simulink model "mrefrobotarm_previous_y_previous_u_previous_ref_cex_2"  (R2018b)
settings: Solver=FixedStepAuto  StartTime=0.0  StopTime=20  RelTol=1e-3  AbsTol=1e-6
undefined symbols (not defined in the file or in its folder): cc, options
libraries: neural x462, simulink x2
(part 6 of 18)

== system mrefrobotarm_previous_y_previous_u_previous_ref_cex_2/Feed-Forward Neural Network1/Layer 3/Delays 1 ==
  "p{3}" : Inport  PortDimensions=30
      mask Display: e = 0.06;c1 = [120 230 180]/255;c2 = ([120 230 180]+0)/(256+128);c3 = ([120 230 180]+128)/(256+128);patch([0 1 1 0],[0 0 1 1],c1);patch([0 1 1 1-e 1-e 0+e],[0 0 1 1-e 0+e 0+e],c2);patch([0 0 1 1-e 0+e 0+e],[0 1 1 1-e 1-e 0+e],c3);plot([0 1 1 0 0],[0 0 1 1 0]);
  mux : Mux  Inputs=1
      mask Display: e = 0.06;c1 = [120 150 230]/255;c2 = ([120 150 230]+0)/383;c3 = ([120 150 230]+128)/383;patch([0 1 1 0],[0 0 1 1],c1);patch([0 1 1 1-e 1-e 0+e],[0 0 1 1-e 0+e 0+e],c2);patch([0 0 1 1-e 0+e 0+e],[0 1 1 1-e 1-e 0+e],c3);plot([0 1 1 0 0],[0 0 1 1 0]);disp('Mux')
  "pd{3,2}" : Outport
      mask Display: e = 0.06;c1 = [120 230 180]/255;c2 = ([120 230 180]+0)/(256+128);c3 = ([120 230 180]+128)/(256+128);patch([0 1 1 0],[0 0 1 1],c1);patch([0 1 1 1-e 1-e 0+e],[0 0 1 1-e 0+e 0+e],c2);patch([0 0 1 1-e 0+e 0+e],[0 1 1 1-e 1-e 0+e],c3);plot([0 1 1 0 0],[0 0 1 1 0]);
  wires:
  "p{3}"/1 -> mux/1
  mux/1 -> "pd{3,2}"/1

== system mrefrobotarm_previous_y_previous_u_previous_ref_cex_2/Feed-Forward Neural Network1/Layer 3/LW{3,2} ==
  "ad{3,2}" : Inport  PortDimensions=30
      mask Display: e = 0.06;c1 = [120 230 180]/255;c2 = ([120 230 180]+0)/(256+128);c3 = ([120 230 180]+128)/(256+128);patch([0 1 1 0],[0 0 1 1],c1);patch([0 1 1 1-e 1-e 0+e],[0 0 1 1-e 0+e 0+e],c2);patch([0 0 1 1-e 0+e 0+e],[0 1 1 1-e 1-e 0+e],c3);plot([0 1 1 0 0],[0 0 1 1 0]);
  "IW{3,2}(1,:)'" : Constant  Value=[0.245566465926212396109207247718586586415767669677734375;-0.56322081322037842454619749332778155803680419921875;-0.28991010367060410235495737651945091784000396728515625;0.3869683333504421174353637979947961866855621337890625;0.496517765752567064030387200546101666986942291259765625;-0.320943780837954883988771825897856615483760833740234375;0.0286370319336148211608605862465992686338722705841064453125;-0.15395906619913668489374458658858202397823333740234375;0.51493301451079076525019218024681322276592254638671875;-0.026941881639260277514491548345176852308213710784912109375;-0.05589778476223307424053388103857287205755710601806640625;0.1600136141061642980343293629630352370440959930419921875;-0.2212967731759021561277478440388222225010395050048828125;-0.168090459815553538991395043922238983213901519775390625;-0.4615503546136172641212169764912687242031097412109375;-0.60839853859597503582534727684105746448040008544921875;0.1504483327033876438605375369661487638950347900390625;-0.4073407234202310878146136019495315849781036376953125;0.331316055045982882365507293798145838081836700439453125;-0.1747391852843100945591459094430319964885711669921875;-0.19591165143500910428286942988052032887935638427734375;0.1816474984983245388736605718804639764130115509033203125;0.3783772749804861224021124144201166927814483642578125;0.046857186277910960192638611943038995377719402313232421875;-0.292883801455053660589555875048972666263580322265625;0.480373124807368323541112431485089473426342010498046875;-0.0158594532240923617727457184400918777100741863250732421875;-0.0228072195102398851684899483416302246041595935821533203125;-0.55934110245892210144802447757683694362640380859375;0.2422309302660256846717601320051471702754497528076171875]
      mask Display: e = 0.06;c1 = [120 150 230]/255;c2 = ([120 150 230]+0)/383;c3 = ([120 150 230]+128)/383;patch([0 1 1 0],[0 0 1 1],c1);patch([0 1 1 1-e 1-e 0+e],[0 0 1 1-e 0+e 0+e],c2);patch([0 0 1 1-e 0+e 0+e],[0 1 1 1-e 1-e 0+e],c3);plot([0 1 1 0 0],[0 0 1 1 0]);disp('weights');
  Mux : Mux  Inputs=1
      mask Display: e = 0.06;c1 = [120 150 230]/255;c2 = ([120 150 230]+0)/383;c3 = ([120 150 230]+128)/383;patch([0 1 1 0],[0 0 1 1],c1);patch([0 1 1 1-e 1-e 0+e],[0 0 1 1-e 0+e 0+e],c2);patch([0 0 1 1-e 0+e 0+e],[0 1 1 1-e 1-e 0+e],c3);plot([0 1 1 0 0],[0 0 1 1 0]);disp('Mux');
  dotprod1 : neural/Weight Functions/dotprod
  "lz{3,2}" : Outport
      mask Display: e = 0.06;c1 = [120 230 180]/255;c2 = ([120 230 180]+0)/(256+128);c3 = ([120 230 180]+128)/(256+128);patch([0 1 1 0],[0 0 1 1],c1);patch([0 1 1 1-e 1-e 0+e],[0 0 1 1-e 0+e 0+e],c2);patch([0 0 1 1-e 0+e 0+e],[0 1 1 1-e 1-e 0+e],c3);plot([0 1 1 0 0],[0 0 1 1 0]);
  wires:
  "IW{3,2}(1,:)'"/1 -> dotprod1/1
  "ad{3,2}"/1 -> dotprod1/2
  dotprod1/1 -> Mux/1
  Mux/1 -> "lz{3,2}"/1

== system mrefrobotarm_previous_y_previous_u_previous_ref_cex_2/cex_m1/Layer 1/Delays 1 ==
  "p{1}" : Inport  PortDimensions=10
      mask Display: e = 0.06;c1 = [120 230 180]/255;c2 = ([120 230 180]+0)/(256+128);c3 = ([120 230 180]+128)/(256+128);patch([0 1 1 0],[0 0 1 1],c1);patch([0 1 1 1-e 1-e 0+e],[0 0 1 1-e 0+e 0+e],c2);patch([0 0 1 1-e 0+e 0+e],[0 1 1 1-e 1-e 0+e],c3);plot([0 1 1 0 0],[0 0 1 1 0]);
  mux : Mux  Inputs=1
      mask Display: e = 0.06;c1 = [120 150 230]/255;c2 = ([120 150 230]+0)/383;c3 = ([120 150 230]+128)/383;patch([0 1 1 0],[0 0 1 1],c1);patch([0 1 1 1-e 1-e 0+e],[0 0 1 1-e 0+e 0+e],c2);patch([0 0 1 1-e 0+e 0+e],[0 1 1 1-e 1-e 0+e],c3);plot([0 1 1 0 0],[0 0 1 1 0]);disp('Mux')
  "pd{1,1}" : Outport
      mask Display: e = 0.06;c1 = [120 230 180]/255;c2 = ([120 230 180]+0)/(256+128);c3 = ([120 230 180]+128)/(256+128);patch([0 1 1 0],[0 0 1 1],c1);patch([0 1 1 1-e 1-e 0+e],[0 0 1 1-e 0+e 0+e],c2);patch([0 0 1 1-e 0+e 0+e],[0 1 1 1-e 1-e 0+e],c3);plot([0 1 1 0 0],[0 0 1 1 0]);
  wires:
  "p{1}"/1 -> mux/1
  mux/1 -> "pd{1,1}"/1

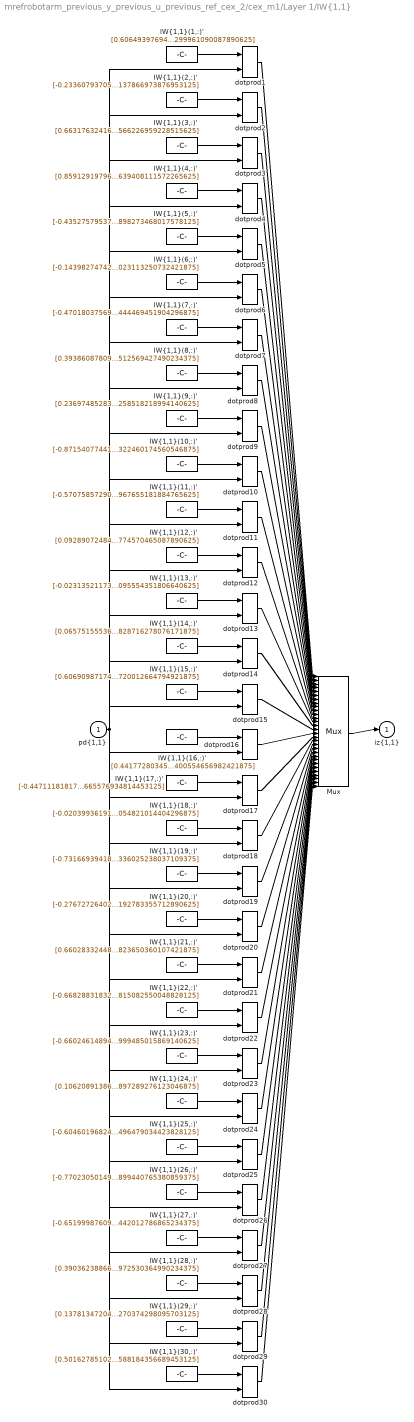
== system mrefrobotarm_previous_y_previous_u_previous_ref_cex_2/cex_m1/Layer 1/IW{1,1} ==
  "pd{1,1}" : Inport  PortDimensions=10
      mask Display: e = 0.06;c1 = [120 230 180]/255;c2 = ([120 230 180]+0)/(256+128);c3 = ([120 230 180]+128)/(256+128);patch([0 1 1 0],[0 0 1 1],c1);patch([0 1 1 1-e 1-e 0+e],[0 0 1 1-e 0+e 0+e],c2);patch([0 0 1 1-e 0+e 0+e],[0 1 1 1-e 1-e 0+e],c3);plot([0 1 1 0 0],[0 0 1 1 0]);
  "IW{1,1}(1,:)'" : Constant  Value=[0.606493976942152013265285859233699738979339599609375;0.300870328462947533854077164505724795162677764892578125;0.58384608162362194860861563938669860363006591796875;-0.183702727789528175161848366769845597445964813232421875;-0.256826958227045765159601842242409475147724151611328125;-0.11957272826138511112592510698959813453257083892822265625;-0.94857591659136308859245900748646818101406097412109375;0.6791329614163685857164409753750078380107879638671875;-0.58145783774079229377917954479926265776157379150390625;0.78323377095806601122518486590706743299961090087890625]
      mask Display: e = 0.06;c1 = [120 150 230]/255;c2 = ([120 150 230]+0)/383;c3 = ([120 150 230]+128)/383;patch([0 1 1 0],[0 0 1 1],c1);patch([0 1 1 1-e 1-e 0+e],[0 0 1 1-e 0+e 0+e],c2);patch([0 0 1 1-e 0+e 0+e],[0 1 1 1-e 1-e 0+e],c3);plot([0 1 1 0 0],[0 0 1 1 0]);disp('Weights');
  "IW{1,1}(10,:)'" : Constant  Value=[-0.87154077441328325903668883256614208221435546875;1.049912196434298561342757238890044391155242919921875;0.27458172096172395182378522804356180131435394287109375;-0.711717329252754549173687337315641343593597412109375;0.27785454353788729964236381420050747692584991455078125;-0.0815691029770375386487302193927462212741374969482421875;0.23890314712288562848385709003196097910404205322265625;0.239853933232654858986876433846191503107547760009765625;-0.62431495878185250258951555224484764039516448974609375;-0.777991313273826090579632364097051322460174560546875]
      mask Display: e = 0.06;c1 = [120 150 230]/255;c2 = ([120 150 230]+0)/383;c3 = ([120 150 230]+128)/383;patch([0 1 1 0],[0 0 1 1],c1);patch([0 1 1 1-e 1-e 0+e],[0 0 1 1-e 0+e 0+e],c2);patch([0 0 1 1-e 0+e 0+e],[0 1 1 1-e 1-e 0+e],c3);plot([0 1 1 0 0],[0 0 1 1 0]);disp('Weights');
  "IW{1,1}(11,:)'" : Constant  Value=[-0.57075857290971854229866266905446536839008331298828125;0.9105044883497910301883848660509102046489715576171875;-0.0274634831225473614868537453048702445812523365020751953125;-0.254607299960154798146305665795807726681232452392578125;-0.2120219789851869596208899793055024929344654083251953125;-0.07760455330727596134909873626384069211781024932861328125;0.42068189247083986881392547729774378240108489990234375;-0.5132735800885883659105957121937535703182220458984375;-0.57046668147494450362700035839225165545940399169921875;-0.750017524258132173287094701663590967655181884765625]
      mask Display: e = 0.06;c1 = [120 150 230]/255;c2 = ([120 150 230]+0)/383;c3 = ([120 150 230]+128)/383;patch([0 1 1 0],[0 0 1 1],c1);patch([0 1 1 1-e 1-e 0+e],[0 0 1 1-e 0+e 0+e],c2);patch([0 0 1 1-e 0+e 0+e],[0 1 1 1-e 1-e 0+e],c3);plot([0 1 1 0 0],[0 0 1 1 0]);disp('Weights');
  "IW{1,1}(12,:)'" : Constant  Value=[0.09289072484482759073376456626647268421947956085205078125;-0.9326730997274779166872349378536455333232879638671875;-0.8047520255107321052179258913383819162845611572265625;-0.530309467610881934973576790071092545986175537109375;0.5676139588165167726430127004277892410755157470703125;-0.60426402156130032405911833848222158849239349365234375;0.416928927700072560202926297279191203415393829345703125;0.56024270477934645651174605518463067710399627685546875;0.130929582458561399871399544281302951276302337646484375;-0.45882086062754334765401154072606004774570465087890625]
      mask Display: e = 0.06;c1 = [120 150 230]/255;c2 = ([120 150 230]+0)/383;c3 = ([120 150 230]+128)/383;patch([0 1 1 0],[0 0 1 1],c1);patch([0 1 1 1-e 1-e 0+e],[0 0 1 1-e 0+e 0+e],c2);patch([0 0 1 1-e 0+e 0+e],[0 1 1 1-e 1-e 0+e],c3);plot([0 1 1 0 0],[0 0 1 1 0]);disp('Weights');
  "IW{1,1}(13,:)'" : Constant  Value=[-0.0231352117399873831449230721091225859709084033966064453125;-0.796505407556588718165357931866310536861419677734375;-0.5816665559413660702148263226263225078582763671875;-0.9505142528724146444574216729961335659027099609375;0.1164862638332339328517406329410732723772525787353515625;0.608926424961647949629650611313991248607635498046875;-0.257541098890456565673190425513894297182559967041015625;0.33512401139020220330877464220975525677204132080078125;0.03018497961469925050526086351965204812586307525634765625;-0.9364213635540326041706293835886754095554351806640625]
      mask Display: e = 0.06;c1 = [120 150 230]/255;c2 = ([120 150 230]+0)/383;c3 = ([120 150 230]+128)/383;patch([0 1 1 0],[0 0 1 1],c1);patch([0 1 1 1-e 1-e 0+e],[0 0 1 1-e 0+e 0+e],c2);patch([0 0 1 1-e 0+e 0+e],[0 1 1 1-e 1-e 0+e],c3);plot([0 1 1 0 0],[0 0 1 1 0]);disp('Weights');
  "IW{1,1}(14,:)'" : Constant  Value=[0.06575155536450284776694985566791729070246219635009765625;-0.99234351852335211940925319140660576522350311279296875;-0.0584833978458139114309233264066278934478759765625;0.157791463982731972048867419289308600127696990966796875;-0.208312265611119429298270233630319125950336456298828125;0.2878455117467508816986310193897224962711334228515625;0.55837583914950694730094937767717055976390838623046875;0.58458401464640552536167206199024803936481475830078125;-0.42939867442946866304964714800007641315460205078125;-0.6031102403934667233187383317272178828716278076171875]
      mask Display: e = 0.06;c1 = [120 150 230]/255;c2 = ([120 150 230]+0)/383;c3 = ([120 150 230]+128)/383;patch([0 1 1 0],[0 0 1 1],c1);patch([0 1 1 1-e 1-e 0+e],[0 0 1 1-e 0+e 0+e],c2);patch([0 0 1 1-e 0+e 0+e],[0 1 1 1-e 1-e 0+e],c3);plot([0 1 1 0 0],[0 0 1 1 0]);disp('Weights');
  "IW{1,1}(15,:)'" : Constant  Value=[0.60690987174474575471805337656405754387378692626953125;0.714888293602866209397461716434918344020843505859375;-0.359764071721432099337789622950367629528045654296875;-0.005782116184957664974108926259077634313143789768218994140625;0.03349733474098283425579580807607271708548069000244140625;0.398232423442965555171468849948723800480365753173828125;0.445672845621305324659289226474356837570667266845703125;-0.5940418562425475723642875891528092324733734130859375;-0.5172060254184474015204386887489818036556243896484375;0.58219671342312562245524532045237720012664794921875]
      mask Display: e = 0.06;c1 = [120 150 230]/255;c2 = ([120 150 230]+0)/383;c3 = ([120 150 230]+128)/383;patch([0 1 1 0],[0 0 1 1],c1);patch([0 1 1 1-e 1-e 0+e],[0 0 1 1-e 0+e 0+e],c2);patch([0 0 1 1-e 0+e 0+e],[0 1 1 1-e 1-e 0+e],c3);plot([0 1 1 0 0],[0 0 1 1 0]);disp('Weights');
  "IW{1,1}(16,:)'" : Constant  Value=[0.441772803454993923111260301084257662296295166015625;-0.858350572502098341232112943544052541255950927734375;0.496601956509376385451304258822347037494182586669921875;0.24716027869555079465868629995384253561496734619140625;0.59088583214640089114055854224716313183307647705078125;0.051540021640639747946277537948844837956130504608154296875;0.89470238214687280997594598375144414603710174560546875;-0.494763825843809346149981820417451672255992889404296875;-0.361008924149344545551088003776385448873043060302734375;-0.46706553192419952846847763794357888400554656982421875]
      mask Display: e = 0.06;c1 = [120 150 230]/255;c2 = ([120 150 230]+0)/383;c3 = ([120 150 230]+128)/383;patch([0 1 1 0],[0 0 1 1],c1);patch([0 1 1 1-e 1-e 0+e],[0 0 1 1-e 0+e 0+e],c2);patch([0 0 1 1-e 0+e 0+e],[0 1 1 1-e 1-e 0+e],c3);plot([0 1 1 0 0],[0 0 1 1 0]);disp('Weights');
  "IW{1,1}(17,:)'" : Constant  Value=[-0.44711181817855483178192343984846957027912139892578125;0.190527695335109215069024912736495025455951690673828125;-0.55197786751330857324404632890946231782436370849609375;0.427144243883912422266035946449846960604190826416015625;0.142254896759542448503310652085929177701473236083984375;-0.863093958059781840574942179955542087554931640625;-0.25772915801204832053628024368663318455219268798828125;0.59760076519626637026050275380839593708515167236328125;0.384121306495605996378372992694494314491748809814453125;0.97143886508737342655450675010797567665576934814453125]
      mask Display: e = 0.06;c1 = [120 150 230]/255;c2 = ([120 150 230]+0)/383;c3 = ([120 150 230]+128)/383;patch([0 1 1 0],[0 0 1 1],c1);patch([0 1 1 1-e 1-e 0+e],[0 0 1 1-e 0+e 0+e],c2);patch([0 0 1 1-e 0+e 0+e],[0 1 1 1-e 1-e 0+e],c3);plot([0 1 1 0 0],[0 0 1 1 0]);disp('Weights');
  "IW{1,1}(18,:)'" : Constant  Value=[-0.0203993619167109306589136252796379267238080501556396484375;0.06789612519323921790981302137879538349807262420654296875;-0.83196043575496381183853600305155850946903228759765625;-0.5780104563247150384341921380837447941303253173828125;0.8767926850877263422745500065502710640430450439453125;0.8984904602706504928022468448034487664699554443359375;-0.29683887374018247395923708609188906848430633544921875;0.53511267268491113924255841993726789951324462890625;0.3149223423667866228470302303321659564971923828125;-0.50917796768627265890927446889691054821014404296875]
      mask Display: e = 0.06;c1 = [120 150 230]/255;c2 = ([120 150 230]+0)/383;c3 = ([120 150 230]+128)/383;patch([0 1 1 0],[0 0 1 1],c1);patch([0 1 1 1-e 1-e 0+e],[0 0 1 1-e 0+e 0+e],c2);patch([0 0 1 1-e 0+e 0+e],[0 1 1 1-e 1-e 0+e],c3);plot([0 1 1 0 0],[0 0 1 1 0]);disp('Weights');
  "IW{1,1}(19,:)'" : Constant  Value=[-0.731669394187537402984844447928480803966522216796875;-0.426830008668516336367559915743186138570308685302734375;-0.65946739269333198851796851158724166452884674072265625;0.3121061831703058064846345587284304201602935791015625;0.0708721051144367286678260597909684292972087860107421875;0.79043143683743510852224289919831790030002593994140625;0.218410546486021039935820908794994466006755828857421875;0.91115469798575166038290262804366648197174072265625;-0.287497511040923026115478933206759393215179443359375;0.484990079632247661489685697233653627336025238037109375]
      mask Display: e = 0.06;c1 = [120 150 230]/255;c2 = ([120 150 230]+0)/383;c3 = ([120 150 230]+128)/383;patch([0 1 1 0],[0 0 1 1],c1);patch([0 1 1 1-e 1-e 0+e],[0 0 1 1-e 0+e 0+e],c2);patch([0 0 1 1-e 0+e 0+e],[0 1 1 1-e 1-e 0+e],c3);plot([0 1 1 0 0],[0 0 1 1 0]);disp('Weights');
  "IW{1,1}(2,:)'" : Constant  Value=[-0.2336079370532533061588509326611529104411602020263671875;-0.74607220811093544199366078828461468219757080078125;-0.369936115928706843458684261349844746291637420654296875;0.45312034973429593520677371998317539691925048828125;0.31261874665209099521945290689473040401935577392578125;0.237541127989350731031237273782608099281787872314453125;-0.8152355017230110689752109465189278125762939453125;1.111565148090730037466755675268359482288360595703125;0.43513570839066917361748210169025696814060211181640625;0.159352016878887781103912857361137866973876953125]
      mask Display: e = 0.06;c1 = [120 150 230]/255;c2 = ([120 150 230]+0)/383;c3 = ([120 150 230]+128)/383;patch([0 1 1 0],[0 0 1 1],c1);patch([0 1 1 1-e 1-e 0+e],[0 0 1 1-e 0+e 0+e],c2);patch([0 0 1 1-e 0+e 0+e],[0 1 1 1-e 1-e 0+e],c3);plot([0 1 1 0 0],[0 0 1 1 0]);disp('Weights');
  "IW{1,1}(20,:)'" : Constant  Value=[-0.276727264025024177751532761249109171330928802490234375;0.6936559254367253846140783934970386326313018798828125;-0.444634416231500406713195161501062102615833282470703125;-0.11718802204525229082587856055397423915565013885498046875;0.601859358495030249969204305671155452728271484375;-1.03049302685429555737073314958252012729644775390625;0.5410489992010465432059618251514621078968048095703125;0.1496380763310218020567532448694691993296146392822265625;-0.25033186406012841729307183413766324520111083984375;-0.69038381027868533923452787348651327192783355712890625]
      mask Display: e = 0.06;c1 = [120 150 230]/255;c2 = ([120 150 230]+0)/383;c3 = ([120 150 230]+128)/383;patch([0 1 1 0],[0 0 1 1],c1);patch([0 1 1 1-e 1-e 0+e],[0 0 1 1-e 0+e 0+e],c2);patch([0 0 1 1-e 0+e 0+e],[0 1 1 1-e 1-e 0+e],c3);plot([0 1 1 0 0],[0 0 1 1 0]);disp('Weights');
  "IW{1,1}(21,:)'" : Constant  Value=[0.66028332448247006869479491797392256557941436767578125;0.2059822140191449324486683281065779738128185272216796875;0.899200650787616684311842618626542389392852783203125;0.1459736644101612135226986310954089276492595672607421875;-0.55273387309170718406647893061744980514049530029296875;-0.376268950753605169179394351886003278195858001708984375;-0.480119058828673839212086704719695262610912322998046875;-0.51806865664255929981862891509081237018108367919921875;-0.86504281608049715668329326945240609347820281982421875;-0.5295864736332098754445496524567715823650360107421875]
      mask Display: e = 0.06;c1 = [120 150 230]/255;c2 = ([120 150 230]+0)/383;c3 = ([120 150 230]+128)/383;patch([0 1 1 0],[0 0 1 1],c1);patch([0 1 1 1-e 1-e 0+e],[0 0 1 1-e 0+e 0+e],c2);patch([0 0 1 1-e 0+e 0+e],[0 1 1 1-e 1-e 0+e],c3);plot([0 1 1 0 0],[0 0 1 1 0]);disp('Weights');
  "IW{1,1}(22,:)'" : Constant  Value=[-0.668288318324803842784831431345082819461822509765625;0.58606698478578334032818020205013453960418701171875;-0.13594007774983574154958887447719462215900421142578125;0.64573069982773312336377102838014252483844757080078125;-0.5683631550204335525222631986252963542938232421875;-0.383970129404375859483167232610867358744144439697265625;-0.34455003807668826976140508122625760734081268310546875;-0.300566767455479888493385942638269625604152679443359375;-0.84771592225582514945614320822642184793949127197265625;0.01101442760038507003017560492708071251399815082550048828125]
      mask Display: e = 0.06;c1 = [120 150 230]/255;c2 = ([120 150 230]+0)/383;c3 = ([120 150 230]+128)/383;patch([0 1 1 0],[0 0 1 1],c1);patch([0 1 1 1-e 1-e 0+e],[0 0 1 1-e 0+e 0+e],c2);patch([0 0 1 1-e 0+e 0+e],[0 1 1 1-e 1-e 0+e],c3);plot([0 1 1 0 0],[0 0 1 1 0]);disp('Weights');
  "IW{1,1}(23,:)'" : Constant  Value=[-0.6602461489436530772678679568343795835971832275390625;0.889022741699142304838687778101302683353424072265625;-0.73775376426502836668674945030943490564823150634765625;0.473046623740375593580864688192377798259258270263671875;0.5896330811756176348836788747576065361499786376953125;-0.126488745698363824754295592356356792151927947998046875;0.276088496086801471474103664149879477918148040771484375;-0.259379579423001771498746848010341636836528778076171875;0.53444578930811059702676857341430149972438812255859375;-0.4517849284879320581609363216557539999485015869140625]
      mask Display: e = 0.06;c1 = [120 150 230]/255;c2 = ([120 150 230]+0)/383;c3 = ([120 150 230]+128)/383;patch([0 1 1 0],[0 0 1 1],c1);patch([0 1 1 1-e 1-e 0+e],[0 0 1 1-e 0+e 0+e],c2);patch([0 0 1 1-e 0+e 0+e],[0 1 1 1-e 1-e 0+e],c3);plot([0 1 1 0 0],[0 0 1 1 0]);disp('Weights');
  "IW{1,1}(24,:)'" : Constant  Value=[0.10620891386625903873852649894615751691162586212158203125;-0.09540789241758608485444170810296782292425632476806640625;-0.67419619035896338754554335537250153720378875732421875;-0.71870519646572772476389445728273130953311920166015625;-1.142330411170607629145479222643189132213592529296875;0.8653091252141196232372521990328095853328704833984375;0.15644385247543024508587450327468104660511016845703125;0.32335968378846347004440531236468814313411712646484375;0.0045070515141347224086221245897831977345049381256103515625;0.11659909305668307577530384833153220824897289276123046875]
      mask Display: e = 0.06;c1 = [120 150 230]/255;c2 = ([120 150 230]+0)/383;c3 = ([120 150 230]+128)/383;patch([0 1 1 0],[0 0 1 1],c1);patch([0 1 1 1-e 1-e 0+e],[0 0 1 1-e 0+e 0+e],c2);patch([0 0 1 1-e 0+e 0+e],[0 1 1 1-e 1-e 0+e],c3);plot([0 1 1 0 0],[0 0 1 1 0]);disp('Weights');
  "IW{1,1}(25,:)'" : Constant  Value=[-0.60460196824824041783585926168598234653472900390625;-0.312658879372127385121160614289692603051662445068359375;0.753970254047653387630134602659381926059722900390625;-0.179249744031663882370963847279199399054050445556640625;-1.01841810925551623512319565634243190288543701171875;-0.577597508590222741275965745444409549236297607421875;0.3688592723785160121252602039021439850330352783203125;0.190224013915391954032685362108168192207813262939453125;-0.2397352610482046120221610863154637627303600311279296875;0.7138221705953740059413803464849479496479034423828125]
      mask Display: e = 0.06;c1 = [120 150 230]/255;c2 = ([120 150 230]+0)/383;c3 = ([120 150 230]+128)/383;patch([0 1 1 0],[0 0 1 1],c1);patch([0 1 1 1-e 1-e 0+e],[0 0 1 1-e 0+e 0+e],c2);patch([0 0 1 1-e 0+e 0+e],[0 1 1 1-e 1-e 0+e],c3);plot([0 1 1 0 0],[0 0 1 1 0]);disp('Weights');
  "IW{1,1}(26,:)'" : Constant  Value=[-0.77023050149346838910702217617654241621494293212890625;-0.89222534152405919005701662172214128077030181884765625;-0.6780355459550484464870123701984994113445281982421875;0.5629607706542409939487470182939432561397552490234375;0.27796985803382623370083592817536555230617523193359375;-0.3021587117833945956846264380146749317646026611328125;0.60181786155237049218413858397980220615863800048828125;0.10816097130853609409317783729420625604689121246337890625;0.26954905191897060579009348657564260065555572509765625;-0.551606447781080699854783233604393899440765380859375]
      mask Display: e = 0.06;c1 = [120 150 230]/255;c2 = ([120 150 230]+0)/383;c3 = ([120 150 230]+128)/383;patch([0 1 1 0],[0 0 1 1],c1);patch([0 1 1 1-e 1-e 0+e],[0 0 1 1-e 0+e 0+e],c2);patch([0 0 1 1-e 0+e 0+e],[0 1 1 1-e 1-e 0+e],c3);plot([0 1 1 0 0],[0 0 1 1 0]);disp('Weights');
  "IW{1,1}(27,:)'" : Constant  Value=[-0.6519998760935272752448099708999507129192352294921875;0.173407039743700697176365110863116569817066192626953125;0.94078390066238692934774690002086572349071502685546875;-0.92705846805173564018076604043017141520977020263671875;-0.457863664540316406270648030840675346553325653076171875;-0.189799580474929285855978378094732761383056640625;0.2446079121309513160209547777412808500230312347412109375;-0.07518343455340907588446697218387271277606487274169921875;0.63856116306209098620882969044032506644725799560546875;-0.299979539069107070670128223355277441442012786865234375]
      mask Display: e = 0.06;c1 = [120 150 230]/255;c2 = ([120 150 230]+0)/383;c3 = ([120 150 230]+128)/383;patch([0 1 1 0],[0 0 1 1],c1);patch([0 1 1 1-e 1-e 0+e],[0 0 1 1-e 0+e 0+e],c2);patch([0 0 1 1-e 0+e 0+e],[0 1 1 1-e 1-e 0+e],c3);plot([0 1 1 0 0],[0 0 1 1 0]);disp('Weights');
  "IW{1,1}(28,:)'" : Constant  Value=[0.39036238866563544025467535902862437069416046142578125;-0.866107533518275740647140992223285138607025146484375;-0.37920335322576936842864370191819034516811370849609375;0.72762816795606155562126104996423237025737762451171875;0.429725443825681174825348307422245852649211883544921875;-0.1885110229048201080370716908873873762786388397216796875;0.7578992069686771859693408259772695600986480712890625;-0.442925105756600434592229476038482971489429473876953125;0.75852426403795103482252670801244676113128662109375;-0.618424967124408198060336872003972530364990234375]
      mask Display: e = 0.06;c1 = [120 150 230]/255;c2 = ([120 150 230]+0)/383;c3 = ([120 150 230]+128)/383;patch([0 1 1 0],[0 0 1 1],c1);patch([0 1 1 1-e 1-e 0+e],[0 0 1 1-e 0+e 0+e],c2);patch([0 0 1 1-e 0+e 0+e],[0 1 1 1-e 1-e 0+e],c3);plot([0 1 1 0 0],[0 0 1 1 0]);disp('Weights');
  "IW{1,1}(29,:)'" : Constant  Value=[0.137813472046091567424497270621941424906253814697265625;0.415202961595532327176982789751491509377956390380859375;0.442724775519893254394077075630775652825832366943359375;0.579194546259369946739070655894465744495391845703125;-0.409135582078520021465095624080277048051357269287109375;-0.2152787159925357574064008758796262554824352264404296875;-0.274764299423147118073273986738058738410472869873046875;-0.77989614816167940336555375324678607285022735595703125;0.74303624657312983270429640469956211745738983154296875;0.82149130359615885055291073513217270374298095703125]
      mask Display: e = 0.06;c1 = [120 150 230]/255;c2 = ([120 150 230]+0)/383;c3 = ([120 150 230]+128)/383;patch([0 1 1 0],[0 0 1 1],c1);patch([0 1 1 1-e 1-e 0+e],[0 0 1 1-e 0+e 0+e],c2);patch([0 0 1 1-e 0+e 0+e],[0 1 1 1-e 1-e 0+e],c3);plot([0 1 1 0 0],[0 0 1 1 0]);disp('Weights');
  "IW{1,1}(3,:)'" : Constant  Value=[0.66317632416791905125563744149985723197460174560546875;-0.1417010585581097437124498128468985669314861297607421875;-0.80664871633892920588237984702573157846927642822265625;0.69365490782746752618237451315508224070072174072265625;0.329870503314372010006394475567503832280635833740234375;-0.5013326646946776321556171751581132411956787109375;-0.2135210148252657536005472138640470802783966064453125;-0.939331354465514412055426873848773539066314697265625;-0.457354096616966077082366837203153409063816070556640625;-0.2222539093961243550356954301605583168566226959228515625]
      mask Display: e = 0.06;c1 = [120 150 230]/255;c2 = ([120 150 230]+0)/383;c3 = ([120 150 230]+128)/383;patch([0 1 1 0],[0 0 1 1],c1);patch([0 1 1 1-e 1-e 0+e],[0 0 1 1-e 0+e 0+e],c2);patch([0 0 1 1-e 0+e 0+e],[0 1 1 1-e 1-e 0+e],c3);plot([0 1 1 0 0],[0 0 1 1 0]);disp('Weights');
  "IW{1,1}(30,:)'" : Constant  Value=[0.5016278510212071051199700377765111625194549560546875;-0.688232005979533933981429072446189820766448974609375;-0.2231614243595181068524624379278975538909435272216796875;-0.53216282502693257328019171836785972118377685546875;0.71568805688240122453436242722091265022754669189453125;-0.2315703822165097458540827801698469556868076324462890625;-0.319117483107429933397725108079612255096435546875;-0.3312151574785964225355883172596804797649383544921875;-0.29772750515552781624961653506034053862094879150390625;-0.7294795423784325993921129338559694588184356689453125]
      mask Display: e = 0.06;c1 = [120 150 230]/255;c2 = ([120 150 230]+0)/383;c3 = ([120 150 230]+128)/383;patch([0 1 1 0],[0 0 1 1],c1);patch([0 1 1 1-e 1-e 0+e],[0 0 1 1-e 0+e 0+e],c2);patch([0 0 1 1-e 0+e 0+e],[0 1 1 1-e 1-e 0+e],c3);plot([0 1 1 0 0],[0 0 1 1 0]);disp('Weights');
  "IW{1,1}(4,:)'" : Constant  Value=[0.85912919796272479988630266234395094215869903564453125;-0.2008483665458993538965870584434014745056629180908203125;-0.6011604443433873345981055535958148539066314697265625;0.37208620439528206080836980618187226355075836181640625;0.6520927171128629851182267884723842144012451171875;-0.60490325453962412449726571139763109385967254638671875;0.7194640156906266792447013358469121158123016357421875;-0.728427830431479517159232273115776479244232177734375;-0.319354767006169826260020272457040846347808837890625;-0.5685341146583002824854702339507639408111572265625]
      mask Display: e = 0.06;c1 = [120 150 230]/255;c2 = ([120 150 230]+0)/383;c3 = ([120 150 230]+128)/383;patch([0 1 1 0],[0 0 1 1],c1);patch([0 1 1 1-e 1-e 0+e],[0 0 1 1-e 0+e 0+e],c2);patch([0 0 1 1-e 0+e 0+e],[0 1 1 1-e 1-e 0+e],c3);plot([0 1 1 0 0],[0 0 1 1 0]);disp('Weights');
  "IW{1,1}(5,:)'" : Constant  Value=[-0.43527579537075478111063375763478688895702362060546875;-0.60808630200562419076959486119449138641357421875;-0.200260709048615426208783674155711196362972259521484375;0.60574859612918874329778873288887552917003631591796875;0.484331051033502657521268019991111941635608673095703125;0.051671150908028880277544914179088664241135120391845703125;-0.6583312723083192263828777868184261023998260498046875;0.11421766706476714492435320380536722950637340545654296875;1.0423563063393199712436398840509355068206787109375;-0.2084679715525341869852837817234103567898273468017578125]
      mask Display: e = 0.06;c1 = [120 150 230]/255;c2 = ([120 150 230]+0)/383;c3 = ([120 150 230]+128)/383;patch([0 1 1 0],[0 0 1 1],c1);patch([0 1 1 1-e 1-e 0+e],[0 0 1 1-e 0+e 0+e],c2);patch([0 0 1 1-e 0+e 0+e],[0 1 1 1-e 1-e 0+e],c3);plot([0 1 1 0 0],[0 0 1 1 0]);disp('Weights');
  "IW{1,1}(6,:)'" : Constant  Value=[-0.14398274742713901286350619557197205722332000732421875;-0.293850299654682178829290251087513752281665802001953125;0.60692347987456785052273744440753944218158721923828125;-0.85037648729738979369585649692453444004058837890625;-0.406544191994274328738612211964209564030170440673828125;-0.4965740649094445569033950960147194564342498779296875;0.9154225429807738567689057163079269230365753173828125;0.09488677668390647912399771257696556858718395233154296875;-0.65305231952250830662620728617184795439243316650390625;-0.425955497888698964015219416978652589023113250732421875]
      mask Display: e = 0.06;c1 = [120 150 230]/255;c2 = ([120 150 230]+0)/383;c3 = ([120 150 230]+128)/383;patch([0 1 1 0],[0 0 1 1],c1);patch([0 1 1 1-e 1-e 0+e],[0 0 1 1-e 0+e 0+e],c2);patch([0 0 1 1-e 0+e 0+e],[0 1 1 1-e 1-e 0+e],c3);plot([0 1 1 0 0],[0 0 1 1 0]);disp('Weights');
  "IW{1,1}(7,:)'" : Constant  Value=[-0.470180375697507646481909659996745176613330841064453125;0.67923253463658994633078691549599170684814453125;0.253031644322486648501779882280970923602581024169921875;0.7482512602499078457896075633470900356769561767578125;0.6403904721837661018213339048088528215885162353515625;-0.29814094449753947291270606001489795744419097900390625;-0.8772235409354520729863224914879538118839263916015625;0.463218090908557533769140945878461934626102447509765625;-0.03631948501986968780297360126496641896665096282958984375;-0.847702107306591567947862131404690444469451904296875]
      mask Display: e = 0.06;c1 = [120 150 230]/255;c2 = ([120 150 230]+0)/383;c3 = ([120 150 230]+128)/383;patch([0 1 1 0],[0 0 1 1],c1);patch([0 1 1 1-e 1-e 0+e],[0 0 1 1-e 0+e 0+e],c2);patch([0 0 1 1-e 0+e 0+e],[0 1 1 1-e 1-e 0+e],c3);plot([0 1 1 0 0],[0 0 1 1 0]);disp('Weights');
  "IW{1,1}(8,:)'" : Constant  Value=[0.39386087809624903410821161742205731570720672607421875;-0.2254268976691275738755138036140124313533306121826171875;0.60184249122802702114398698540753684937953948974609375;0.9230867323841749350066265833447687327861785888671875;-0.431888000865165044839244501417852006852626800537109375;0.467412984879591208997595686014392413198947906494140625;0.186226157488242394233424192862003110349178314208984375;-0.1574227693649177250989623644272796809673309326171875;0.6284979822048122333200126377050764858722686767578125;-0.1370603342838430105388169977231882512569427490234375]
      mask Display: e = 0.06;c1 = [120 150 230]/255;c2 = ([120 150 230]+0)/383;c3 = ([120 150 230]+128)/383;patch([0 1 1 0],[0 0 1 1],c1);patch([0 1 1 1-e 1-e 0+e],[0 0 1 1-e 0+e 0+e],c2);patch([0 0 1 1-e 0+e 0+e],[0 1 1 1-e 1-e 0+e],c3);plot([0 1 1 0 0],[0 0 1 1 0]);disp('Weights');
  "IW{1,1}(9,:)'" : Constant  Value=[0.2369748528362038142436318821637541987001895904541015625;-0.1681523495018608926887537791117210872471332550048828125;0.11313514708015910692484595756468479521572589874267578125;-0.481734972986217979684653300864738412201404571533203125;0.9380193810788355346375055887619964778423309326171875;-0.79013428439663668800818641102523542940616607666015625;-0.58036992174079726769519993467838503420352935791015625;-0.651961957489657351061396184377372264862060546875;0.06918641538627057219201788029749877750873565673828125;0.55250492850610799511201776113011874258518218994140625]
      mask Display: e = 0.06;c1 = [120 150 230]/255;c2 = ([120 150 230]+0)/383;c3 = ([120 150 230]+128)/383;patch([0 1 1 0],[0 0 1 1],c1);patch([0 1 1 1-e 1-e 0+e],[0 0 1 1-e 0+e 0+e],c2);patch([0 0 1 1-e 0+e 0+e],[0 1 1 1-e 1-e 0+e],c3);plot([0 1 1 0 0],[0 0 1 1 0]);disp('Weights');
  Mux : Mux  Inputs=30
      mask Display: e = 0.06;c1 = [120 150 230]/255;c2 = ([120 150 230]+0)/383;c3 = ([120 150 230]+128)/383;patch([0 1 1 0],[0 0 1 1],c1);patch([0 1 1 1-e 1-e 0+e],[0 0 1 1-e 0+e 0+e],c2);patch([0 0 1 1-e 0+e 0+e],[0 1 1 1-e 1-e 0+e],c3);plot([0 1 1 0 0],[0 0 1 1 0]);disp('Mux');
  dotprod{1..30} (30 alike) : neural/Weight Functions/dotprod
  "iz{1,1}" : Outport
      mask Display: e = 0.06;c1 = [120 230 180]/255;c2 = ([120 230 180]+0)/(256+128);c3 = ([120 230 180]+128)/(256+128);patch([0 1 1 0],[0 0 1 1],c1);patch([0 1 1 1-e 1-e 0+e],[0 0 1 1-e 0+e 0+e],c2);patch([0 0 1 1-e 0+e 0+e],[0 1 1 1-e 1-e 0+e],c3);plot([0 1 1 0 0],[0 0 1 1 0]);
  wires:
  "IW{1,1}(1,:)'"/1 -> dotprod1/1
  "pd{1,1}"/1 -> dotprod1/2, dotprod2/2, dotprod3/2, dotprod4/2, dotprod5/2, dotprod6/2, dotprod7/2, dotprod8/2, dotprod9/2, dotprod10/2, dotprod11/2, dotprod12/2, dotprod13/2, dotprod14/2, dotprod15/2, dotprod16/2, dotprod17/2, dotprod18/2, dotprod19/2, dotprod20/2, dotprod21/2, dotprod22/2, dotprod23/2, dotprod24/2, dotprod25/2, dotprod26/2, dotprod27/2, dotprod28/2, dotprod29/2, dotprod30/2
  dotprod1/1 -> Mux/1
  "IW{1,1}(2,:)'"/1 -> dotprod2/1
  dotprod2/1 -> Mux/2
  "IW{1,1}(3,:)'"/1 -> dotprod3/1
  dotprod3/1 -> Mux/3
  "IW{1,1}(4,:)'"/1 -> dotprod4/1
  dotprod4/1 -> Mux/4
  "IW{1,1}(5,:)'"/1 -> dotprod5/1
  dotprod5/1 -> Mux/5
  "IW{1,1}(6,:)'"/1 -> dotprod6/1
  dotprod6/1 -> Mux/6
  "IW{1,1}(7,:)'"/1 -> dotprod7/1
  dotprod7/1 -> Mux/7
  "IW{1,1}(8,:)'"/1 -> dotprod8/1
  dotprod8/1 -> Mux/8
  "IW{1,1}(9,:)'"/1 -> dotprod9/1
  dotprod9/1 -> Mux/9
  "IW{1,1}(10,:)'"/1 -> dotprod10/1
  dotprod10/1 -> Mux/10
  "IW{1,1}(11,:)'"/1 -> dotprod11/1
  dotprod11/1 -> Mux/11
  "IW{1,1}(12,:)'"/1 -> dotprod12/1
  dotprod12/1 -> Mux/12
  "IW{1,1}(13,:)'"/1 -> dotprod13/1
  dotprod13/1 -> Mux/13
  "IW{1,1}(14,:)'"/1 -> dotprod14/1
  dotprod14/1 -> Mux/14
  "IW{1,1}(15,:)'"/1 -> dotprod15/1
  dotprod15/1 -> Mux/15
  "IW{1,1}(16,:)'"/1 -> dotprod16/1
  dotprod16/1 -> Mux/16
  "IW{1,1}(17,:)'"/1 -> dotprod17/1
  dotprod17/1 -> Mux/17
  "IW{1,1}(18,:)'"/1 -> dotprod18/1
  dotprod18/1 -> Mux/18
  "IW{1,1}(19,:)'"/1 -> dotprod19/1
  dotprod19/1 -> Mux/19
  "IW{1,1}(20,:)'"/1 -> dotprod20/1
  dotprod20/1 -> Mux/20
  "IW{1,1}(21,:)'"/1 -> dotprod21/1
  dotprod21/1 -> Mux/21
  "IW{1,1}(22,:)'"/1 -> dotprod22/1
  dotprod22/1 -> Mux/22
  "IW{1,1}(23,:)'"/1 -> dotprod23/1
  dotprod23/1 -> Mux/23
  "IW{1,1}(24,:)'"/1 -> dotprod24/1
  dotprod24/1 -> Mux/24
  "IW{1,1}(25,:)'"/1 -> dotprod25/1
  dotprod25/1 -> Mux/25
  "IW{1,1}(26,:)'"/1 -> dotprod26/1
  dotprod26/1 -> Mux/26
  "IW{1,1}(27,:)'"/1 -> dotprod27/1
  dotprod27/1 -> Mux/27
  "IW{1,1}(28,:)'"/1 -> dotprod28/1
  dotprod28/1 -> Mux/28
  "IW{1,1}(29,:)'"/1 -> dotprod29/1
  dotprod29/1 -> Mux/29
  "IW{1,1}(30,:)'"/1 -> dotprod30/1
  dotprod30/1 -> Mux/30
  Mux/1 -> "iz{1,1}"/1

== system mrefrobotarm_previous_y_previous_u_previous_ref_cex_2/cex_m1/Layer 2/Delays 1 ==
  "p{2}" : Inport  PortDimensions=30
      mask Display: e = 0.06;c1 = [120 230 180]/255;c2 = ([120 230 180]+0)/(256+128);c3 = ([120 230 180]+128)/(256+128);patch([0 1 1 0],[0 0 1 1],c1);patch([0 1 1 1-e 1-e 0+e],[0 0 1 1-e 0+e 0+e],c2);patch([0 0 1 1-e 0+e 0+e],[0 1 1 1-e 1-e 0+e],c3);plot([0 1 1 0 0],[0 0 1 1 0]);
  mux : Mux  Inputs=1
      mask Display: e = 0.06;c1 = [120 150 230]/255;c2 = ([120 150 230]+0)/383;c3 = ([120 150 230]+128)/383;patch([0 1 1 0],[0 0 1 1],c1);patch([0 1 1 1-e 1-e 0+e],[0 0 1 1-e 0+e 0+e],c2);patch([0 0 1 1-e 0+e 0+e],[0 1 1 1-e 1-e 0+e],c3);plot([0 1 1 0 0],[0 0 1 1 0]);disp('Mux')
  "pd{2,1}" : Outport
      mask Display: e = 0.06;c1 = [120 230 180]/255;c2 = ([120 230 180]+0)/(256+128);c3 = ([120 230 180]+128)/(256+128);patch([0 1 1 0],[0 0 1 1],c1);patch([0 1 1 1-e 1-e 0+e],[0 0 1 1-e 0+e 0+e],c2);patch([0 0 1 1-e 0+e 0+e],[0 1 1 1-e 1-e 0+e],c3);plot([0 1 1 0 0],[0 0 1 1 0]);
  wires:
  "p{2}"/1 -> mux/1
  mux/1 -> "pd{2,1}"/1
